simulink model "smulaciones_lab1"  (R2024a)
settings: Solver=VariableStepAuto  StartTime=0.0  StopTime=50  RelTol=1e-3
settings Model: Creator=Usuario  LastModifiedBy=Usuario

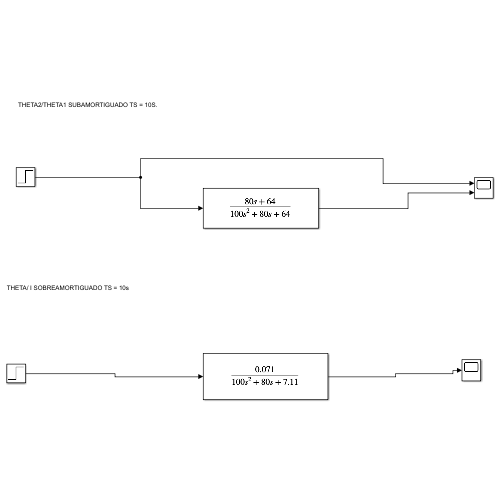
[thumbnail: Simulink's stored preview of the top-level diagram]
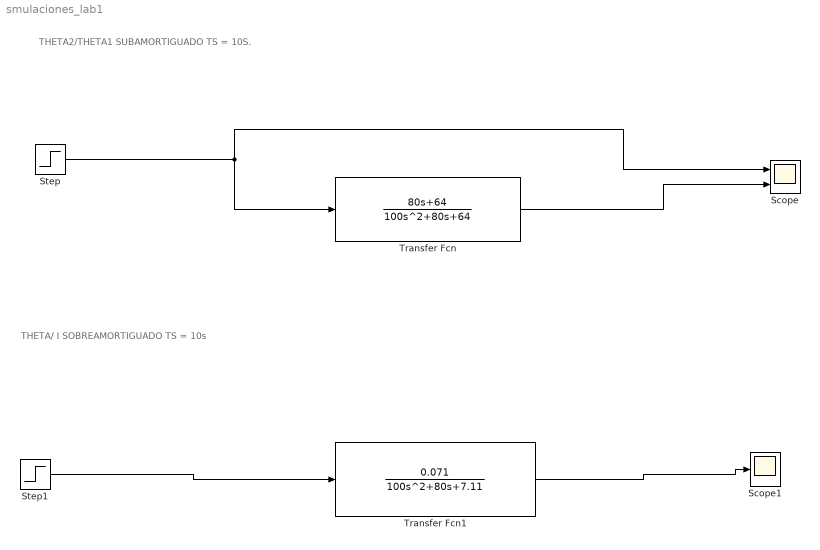
== system smulaciones_lab1 ==
  note: THETA2/THETA1 SUBAMORTIGUADO TS = 10S.
  note: THETA/ I SOBREAMORTIGUADO TS = 10s
  Scope : Scope  NumInputPorts=2
  Scope1 : Scope
  Step : Step  SampleTime=0
  Step1 : Step  SampleTime=0
  Transfer Fcn : TransferFcn  Numerator=[80 64]  Denominator=[100 80 64]
  Transfer Fcn1 : TransferFcn  Numerator=[0.071]  Denominator=[100 80 7.11]
  wires:
  Step/1 -> Transfer Fcn/1, Scope/1
  Transfer Fcn/1 -> Scope/2
  Transfer Fcn1/1 -> Scope1/1
  Step1/1 -> Transfer Fcn1/1
